simulink model "subsystems_saturation"  (R2024b)
settings: Solver=VariableStepAuto  StartTime=0.0  StopTime=10.0  RelTol=1e-3
settings Model: Creator=Ahmad  LastModifiedBy=Ahmad

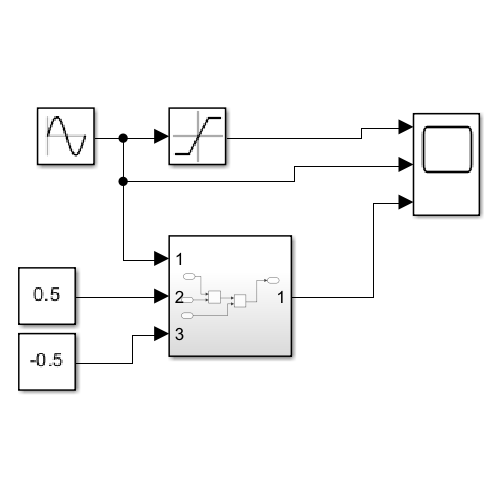
[thumbnail: Simulink's stored preview of the top-level diagram]
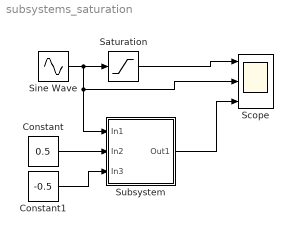
== system subsystems_saturation ==
  Constant : Constant  Value=0.5
  Constant1 : Constant  Value=-0.5
  Saturation : Saturate
  Scope : Scope  NumInputPorts=3
  Sine Wave : Sin  SampleTime=0
  Subsystem : Subsystem
  wires:
  Saturation/1 -> Scope/1
  Sine Wave/1 -> Subsystem/1(In1), Scope/2, Saturation/1
  Constant/1 -> Subsystem/2(In2)
  Constant1/1 -> Subsystem/3(In3)
  Subsystem/1(Out1) -> Scope/3

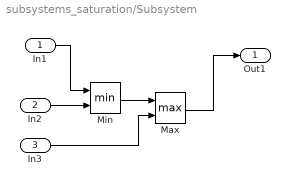
== system subsystems_saturation/Subsystem ==
  In1 : Inport
  In2 : Inport  Port=2
  In3 : Inport  Port=3
  Max : MinMax  Function=max  Inputs=2
  Min : MinMax  Inputs=2
  Out1 : Outport
  wires:
  In1/1 -> Min/1
  Min/1 -> Max/1
  In3/1 -> Max/2
  In2/1 -> Min/2
  Max/1 -> Out1/1
